simulink model "AHRS_Voter_Harness_HLR_11"  (R2026b)
settings: Solver=FixedStepDiscrete  EnableMultiTasking=on
settings Model: DataDictionary=DD_AHRS_Voter.sldd  Creator=The MathWorks, Inc.  LastModifiedBy=The MathWorks, Inc.
settings DataIOCC: InputTimeTolerance=off  LimitDataPoints=on
settings OptimizationCC: BlockReduction=off  DefaultParameterBehavior=Inlined  EfficientFloat2IntCast=on  EfficientMapNaN2IntZero=off  EfficientTunableParamExpr=on  EnhancedBackFolding=on  InlineInvariantSignals=on  LifeSpan=inf  MaxStackSize=inf  OptimizeBlockOrder=speed  PassReuseOutputArgsAs=Individual arguments  UseDivisionForNetSlopeComputation=on  UseFloatMulNetSlope=on
settings DebuggingCC: AlgebraicLoopMsg=error  AllowSymbolicDim=off  ArithmeticOperatorsInVariantConditions=warning  ArtificialAlgebraicLoopMsg=error  AssertControl=DisableAll  BlockPriorityViolationMsg=error  BusObjectLabelMismatch=error  CheckMatrixSingularityMsg=error  InheritedTsInSrcMsg=error  IntegerOverflowMsg=error  IntegerSaturationMsg=error  ModelReferenceDataLoggingMessage=error  ModelReferenceIOMismatchMessage=error  ModelReferenceSymbolNameMessage=none  NonBusSignalsTreatedAsBus=error  ParameterPrecisionLossMsg=error  ParameterTunabilityLossMsg=error  ParameterUnderflowMsg=error  PregeneratedLibrarySubsystemCodeDiagnostic=none  ReadBeforeWriteMsg=EnableAllAsError  RootOutportRequireBusObject=error  SFExecutionAtInitializationDiag=none  SFInvalidInputDataAccessInChartInitDiag=error  SFTransitionActionBeforeConditionDiag=error  SFTransitionOutsideNaturalParentDiag=error  SFUndirectedBroadcastEventsDiag=error  SFUnreachableExecutionPathDiag=error  SFcnCompatibilityMsg=error  SaveWithDisabledLinksMsg=error  SaveWithParameterizedLinksMsg=error  SigSpecEnsureSampleTimeMsg=error  SignalInfNanChecking=error  SignalLabelMismatchMsg=error  SignalRangeChecking=error  SingleTaskRateTransMsg=error  SolverPrmCheckMsg=error  StateNameClashWarn=warning  StrictBusMsg=ErrorOnBusTreatedAsVector  TasksWithSamePriorityMsg=error  UnconnectedInputMsg=error  UnconnectedLineMsg=error  UnconnectedOutputMsg=error  UnderSpecifiedDataTypeMsg=error  UniqueDataStoreMsg=error  UnknownTsInhSupMsg=error  UnnecessaryDatatypeConvMsg=warning  VectorMatrixConversionMsg=error  WriteAfterReadMsg=EnableAllAsError  WriteAfterWriteMsg=EnableAllAsError
settings HardwareCC: ProdHWDeviceType=ARM Compatible->ARM 10  ProdLargestAtomicInteger=Long
settings ModelReferenceCC: ModelReferenceNumInstancesAllowed=Single  PropagateSignalLabelsOutOfModel=off
settings SFSimCC: CustomCodeUndefinedFunction=UseInterfaceOnly  EnableRuntimeRecursion=off  MATLABDynamicMemAlloc=off
settings RTWCC: BuildConfiguration=Faster Runs  DLArmComputeVersion=19.05  Description=Embedded Coder  GenCodeOnly=on  GenerateCodeMetricsReport=on  GenerateReport=on  GenerateTraceInfo=on  GenerateTraceReport=on  GenerateTraceReportEml=on  GenerateTraceReportSf=on  GenerateTraceReportSl=on  IncludeHyperlinkInReport=on  LaunchReport=on  SystemTargetFile=ert.tlc  TemplateMakefile=ert_default_tmf
settings CodeAppCC: ForceParamTrailComments=on  IgnoreCustomStorageClasses=off  MATLABFcnDesc=on  ReqsInCode=on  StateflowObjectComments=on
settings ERTTargetCC: CastingMode=Standards  DynamicArrayContainerType=coder::array  EnableSignedLeftShifts=off  EnableSignedRightShifts=off  GenerateSampleERTMain=on  GenerateSharedConstants=off  IncludeMdlTerminateFcn=off  ParenthesesLevel=Maximum  PreserveExpressionOrder=on  PreserveIfCondition=on  RemoveDisableFunc=on  SubcomponentCodeInterfacePackaging=Nonreusable function  SupportAbsoluteTime=off  SupportNonFinite=off  SuppressErrorStatus=on  UtilityFuncGeneration=Shared location

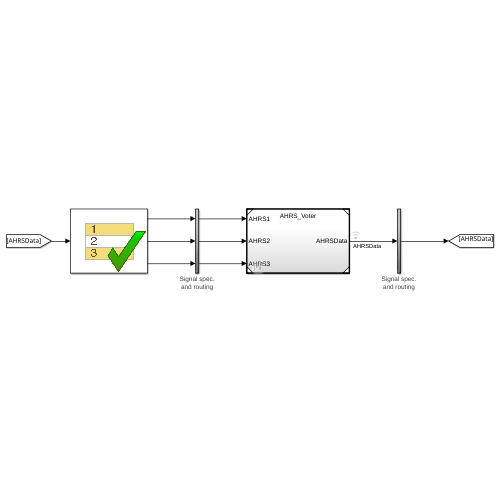
[thumbnail: Simulink's stored preview of the top-level diagram]
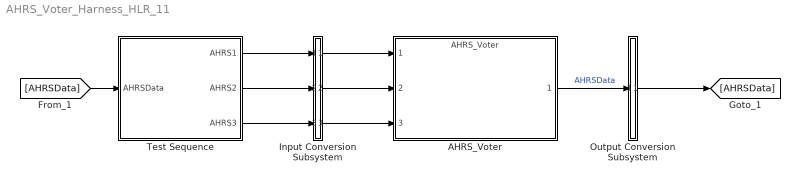
== system AHRS_Voter_Harness_HLR_11 ==
  AHRS_Voter : ModelReference  ModelNameDialog=AHRS_Voter  SimulationMode=Normal  ModelReferenceVersion=7.4
  Input Conversion Subsystem : Subsystem  Tag=__SLT_ICS__  Description=|
      | Signal spec.
      | and routing
      settings: AttributesFormatString=%<Description>
  Output Conversion Subsystem : Subsystem  Tag=__SLT_OCS__  Description=|
      | Signal spec.
      | and routing
      settings: AttributesFormatString=%<Description>
  Test Sequence : Test Sequence  TreatAsAtomicUnit=on
  wires:
  Test Sequence/1(AHRS1) -> Input Conversion Subsystem/1(Inport_1)
  Test Sequence/2(AHRS2) -> Input Conversion Subsystem/2(Inport_2)
  Test Sequence/3(AHRS3) -> Input Conversion Subsystem/3(Inport_3)
  [AHRSData] -> Test Sequence/1(AHRSData)
  Output Conversion Subsystem/1(Outport_1) -> [AHRSData]
  Input Conversion Subsystem/1(Outport_1) -> AHRS_Voter/1
  Input Conversion Subsystem/2(Outport_2) -> AHRS_Voter/2
  Input Conversion Subsystem/3(Outport_3) -> AHRS_Voter/3
  AHRS_Voter/1 -> Output Conversion Subsystem/1(Inport_1)  "AHRSData"

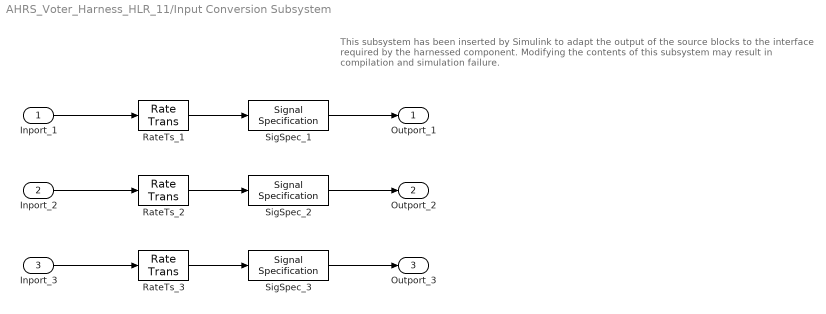
== system AHRS_Voter_Harness_HLR_11/Input Conversion Subsystem ==
  note: This subsystem has been inserted by Simulink to adapt the output of the source blocks to the interface required by the harnessed component.
      |  Modifying the contents of this subsystem may result in compilation and simulation failure.
  Inport_1 : Inport
  Inport_2 : Inport  Port=2
  Inport_3 : Inport  Port=3
  RateTs_1 : RateTransition  OutPortSampleTime=0.01
  RateTs_2 : RateTransition  OutPortSampleTime=0.01
  RateTs_3 : RateTransition  OutPortSampleTime=0.01
  SigSpec_1 : SignalSpecification  OutDataTypeStr=Bus: AHRS_Bus  Dimensions=[1]  SampleTime=0.01  BusOutputAsStruct=on
  SigSpec_2 : SignalSpecification  OutDataTypeStr=Bus: AHRS_Bus  Dimensions=[1]  SampleTime=0.01  BusOutputAsStruct=on
  SigSpec_3 : SignalSpecification  OutDataTypeStr=Bus: AHRS_Bus  Dimensions=[1]  SampleTime=0.01  BusOutputAsStruct=on
  Outport_1 : Outport  VectorParamsAs1DForOutWhenUnconnected=off
  Outport_2 : Outport  Port=2  VectorParamsAs1DForOutWhenUnconnected=off
  Outport_3 : Outport  Port=3  VectorParamsAs1DForOutWhenUnconnected=off
  wires:
  SigSpec_1/1 -> Outport_1/1
  RateTs_1/1 -> SigSpec_1/1
  Inport_1/1 -> RateTs_1/1
  SigSpec_2/1 -> Outport_2/1
  RateTs_2/1 -> SigSpec_2/1
  Inport_2/1 -> RateTs_2/1
  SigSpec_3/1 -> Outport_3/1
  RateTs_3/1 -> SigSpec_3/1
  Inport_3/1 -> RateTs_3/1

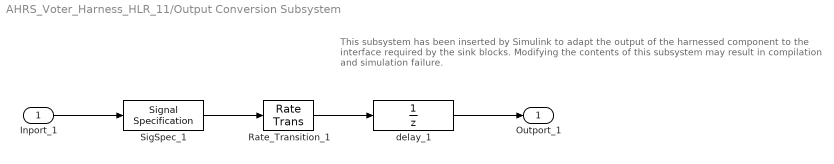
== system AHRS_Voter_Harness_HLR_11/Output Conversion Subsystem ==
  note: This subsystem has been inserted by Simulink to adapt the output of the harnessed component to the interface required by the sink blocks.
      |  Modifying the contents of this subsystem may result in compilation and simulation failure.
  Inport_1 : Inport
  Rate_Transition_1 : RateTransition  OutPortSampleTimeOpt=Inherit
  SigSpec_1 : SignalSpecification  OutDataTypeStr=double  Dimensions=[5]  SampleTime=0.01
  delay_1 : UnitDelay  SampleTime=-1
  Outport_1 : Outport  VectorParamsAs1DForOutWhenUnconnected=off
  wires:
  Inport_1/1 -> SigSpec_1/1
  SigSpec_1/1 -> Rate_Transition_1/1
  Rate_Transition_1/1 -> delay_1/1
  delay_1/1 -> Outport_1/1

== stateflow chart AHRS_Voter_Harness_HLR_11/Test Sequence ==
  state step_0
    %% Initialize data outputs.
    AHRS1.valid = true;
    AHRS1.theta = 0;
    AHRS1.phi = 0;
    AHRS1.r = 0;
    AHRS1.q = 0;
    AHRS1.p = 0;
    AHRS2.valid = true;
    AHRS2.theta = 0;
    AHRS2.phi = 0;
    AHRS2.r = 0;
    AHRS2.q = 0;
    AHRS2.p = 0;
    AHRS3.valid = true;
    AHRS3.theta = 0;
    AHRS3.phi = 0;
    AHRS3.r = 0;
    AHRS3.q = 0;
    AHRS3.p = 0;
  state step_1
    % Test that all outputs are set to zero uisng the tolerance
    verify(abs(AHRSData(1))<Tol, 'HLR11 step_1: Zero output condition failed for theta');
    verify(abs(AHRSData(2))<Tol, 'HLR11 step_1: Zero output condition failed for phi');
    verify(abs(AHRSData(3))<Tol, 'HLR11 step_1: Zero output condition failed for r');
    verify(abs(AHRSData(4))<Tol, 'HLR11 step_1: Zero output condition failed for q');
    verify(abs(AHRSData(5))<Tol, 'HLR11 step_1: Zero output condition failed for p');
  state step_2
    % Set data to different values for each AHRS and each element
    % AHRS1
    AHRS1.theta = 1;
    AHRS1.phi = -2;
    AHRS1.r = 3;
    AHRS1.q = 4;
    AHRS1.p = 0;
    % AHRS2
    AHRS2.theta = -1;
    AHRS2.phi = 2;
    AHRS2.r = -3;
    AHRS2.q = -4;
    AHRS2.p = -5;
    % AHRS3
    AHRS3.theta = 5;
    AHRS3.phi = 4;
    AHRS3.r = 3;
    AHRS3.q = -2;
    AHRS3.p = 1;
  state step_3
    % Test that each element is the mid value, based on the three inputs
    verify((AHRSData(1)-AHRS1.theta)<Tol, 'HLR_11 step_3: Mid value selection failed for AHRS1 theta');
    verify((AHRSData(2)-AHRS2.phi)<Tol, 'HLR_11 step_3: Mid value selection failed for AHRS2 phi');
    verify((AHRSData(3)-AHRS3.r)<Tol, 'HLR_11 step_3: Mid value selection failed for AHRS3 r');
    verify((AHRSData(4)-AHRS3.q)<Tol, 'HLR_11 step_3: Mid value selection failed for AHRS3 q');
    verify((AHRSData(5)-AHRS1.p)<Tol, 'HLR_11 step_3: Mid value selection failed for AHRS1 p');
  state step_4
    % Set data to different vlaues at or near full positive range for each AHRS and each element
    % AHRS1
    AHRS1.theta = 90;
    AHRS1.phi = 179;
    AHRS1.r = 60;
    AHRS1.q = 58;
    AHRS1.p = 58;
    % AHRS2
    AHRS2.theta = 89;
    AHRS2.phi = 180;
    AHRS2.r = 59;
    AHRS2.q = 59;
    AHRS2.p = 60;
    % AHRS3
    AHRS3.theta = 88;
    AHRS3.phi = 178;
    AHRS3.r = 58;
    AHRS3.q = 60;
    AHRS3.p = 59;
  state step_5
    % Test that each element is the mid value, based on the three inputs
    verify((AHRSData(1)-AHRS2.theta)<Tol, 'HLR_11 step_5: Mid value selection failed for AHRS2 theta');
    verify((AHRSData(2)-AHRS1.phi)<Tol, 'HLR_11 step_5: Mid value selection failed for AHRS1 phi');
    verify((AHRSData(3)-AHRS2.r)<Tol, 'HLR_11 step_5: Mid value selection failed for AHRS2 r');
    verify((AHRSData(4)-AHRS2.q)<Tol, 'HLR_11 step_5: Mid value selection failed for AHRS2 q');
    verify((AHRSData(5)-AHRS3.p)<Tol, 'HLR_11 step_5: Mid value selection failed for AHRS3 p');
  state step_6
    % Set data to different vlaues at or near full negative range for each AHRS and each element
    % AHRS1
    AHRS1.theta = -90;
    AHRS1.phi = -178;
    AHRS1.r = -59;
    AHRS1.q = -59;
    AHRS1.p = -60;
    % AHRS2
    AHRS2.theta = -88;
    AHRS2.phi = -180;
    AHRS2.r = -60;
    AHRS2.q = -58;
    AHRS2.p = -59;
    % AHRS3
    AHRS3.theta = -89;
    AHRS3.phi = -179;
    AHRS3.r = -58;
    AHRS3.q = -60;
    AHRS3.p = -58;
  state step_7
    % Test that each element is the mid value, based on the three inputs
    verify((AHRSData(1)-AHRS3.theta)<Tol, 'HLR_11 Step_7: Mid value selection failed for AHRS3 theta');
    verify((AHRSData(2)-AHRS3.phi)<Tol, 'HLR_11 Step_7: Mid value selection failed for AHRS3 phi');
    verify((AHRSData(3)-AHRS1.r)<Tol, 'HLR_11 Step_7: Mid value selection failed for AHRS1 r');
    verify((AHRSData(4)-AHRS1.q)<Tol, 'HLR_11 Step_7: Mid value selection failed for AHRS1 q');
    verify((AHRSData(5)-AHRS2.p)<Tol, 'HLR_11 Step_7: Mid value selection failed for AHRS2 p');
  (default) -> step_0
  step_0 -> step_1 : [after(1, sec)
      | ]
  step_1 -> step_2
  step_2 -> step_3 : [after(1, sec)
      | ]
  step_3 -> step_4
  step_4 -> step_5 : [after(1, sec)
      | ]
  step_5 -> step_6
  step_6 -> step_7 : [after(1, sec)
      | ]
  data: AHRSData input double size=[5]; AHRS1 output Bus: AHRS_Bus size=[1]; AHRS2 output Bus: AHRS_Bus size=[1]; AHRS3 output Bus: AHRS_Bus size=[1]; Tol constant double =1e-7
